simulink model "MPCwithStage"  (R2019b)
settings: Solver=ode8  StartTime=0.0  StopTime=5  RelTol=1e-3
settings Model: Creator=cwh  LastModifiedBy=cwh

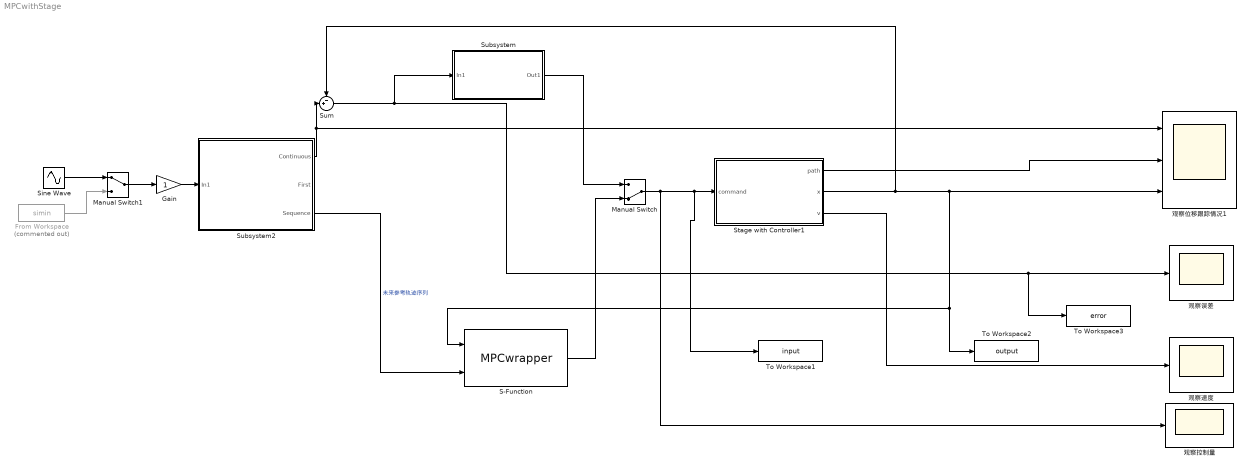
== system MPCwithStage ==
  From Workspace : FromWorkspace  Commented=on  VariableName=simin
  Gain : Gain
  Manual Switch : ManualSwitch  CurrentSetting=0
  Manual Switch1 : ManualSwitch
  S-Function : S-Function  FunctionName=MPCwrapper  Parameters=ts0,p0,m0,wy0,wu0,pn0,mn0,A0,B0,C0  SFunctionDeploymentMode=off  EnableBusSupport=off  mask{ts0=1/300, p0=15, m0=2, wy0=1, wu0=2, pn0=0.01, mn0=1e-7, A0=[1.00001139444525 0.000608242190743377;-0.00132825987534539 0.740443856051726], B0=[0.00434874017606072;-35.613687675832], C0=[-6.04865289015463 -0.00170156787433402]}
      mask Display:
      | fprintf('MyMPCinC++');
      | port_label('input', 1, 'mo')
      | port_label('input', 2, 'ref')
      | port_label('output', 1, 'mv')
  Sine Wave : Sin  Amplitude=0.001  Frequency=2*3.1415926*2  SampleTime=0
  Stage with Controller1 : Subsystem  mask{tc=1/300, ts=5e-5, vm=0.5, am=3}
      mask prompts: tc "Command period"; ts "Servoing period"; vm "vmax"; am "amax"
  Subsystem : Subsystem  mask{kp=2, ki=0, kd=0.01}
      mask Display:
      | fprintf('PID Controller');
      | port_label('input', 1, 'error')
      | port_label('output', 1, 'out')
  Subsystem2 : Subsystem  mask{tc=1/300, p=15}
      mask prompts: tc "Control period"; p "Preview Length"
  Sum : Sum  Inputs=-+|
  To Workspace1 : ToWorkspace  VariableName=input  SampleTime=1/300
      settings: Save2DSignal=2-D array (concatenate along first dimension)
  To Workspace2 : ToWorkspace  VariableName=output  SampleTime=1/300
      settings: Save2DSignal=2-D array (concatenate along first dimension)
  To Workspace3 : ToWorkspace  VariableName=error  SampleTime=1/300
      settings: Save2DSignal=2-D array (concatenate along first dimension)
  观察位移跟踪情况1 : Scope  NumInputPorts=3
  观察控制量 : Scope
  观察误差 : Scope
  观察速度 : Scope
  wires:
  S-Function/1 -> Manual Switch/2
  From Workspace/1 -> Manual Switch1/2
  Gain/1 -> Subsystem2/1(In1)
  Manual Switch1/1 -> Gain/1
  Sine Wave/1 -> Manual Switch1/1
  Subsystem2/3(Sequence) -> S-Function/2  "未来参考轨迹序列"
  Manual Switch/1 -> Stage with Controller1/1(command), To Workspace1/1, 观察控制量/1
  Stage with Controller1/2(x) -> Sum/1, S-Function/1, To Workspace2/1, 观察位移跟踪情况1/3
  Sum/1 -> To Workspace3/1, 观察误差/1, Subsystem/1(In1)
  Stage with Controller1/1(path) -> 观察位移跟踪情况1/2
  Subsystem/1(Out1) -> Manual Switch/1
  Stage with Controller1/3(v) -> 观察速度/1
  Subsystem2/1(Continuous) -> 观察位移跟踪情况1/1, Sum/2

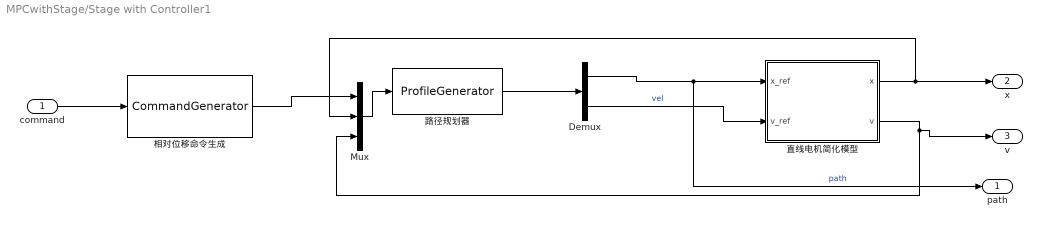
== system MPCwithStage/Stage with Controller1 ==
  command : Inport
  Demux : Demux  Outputs=2
  Mux : Mux  Inputs=3
  直线电机简化模型 : Subsystem  mask{ts=ts, L=1.94e-3, R=2.46, Ki=4.6, Kf=0, Kbemf=2.81, M=1, Kpx=15, Kix=0.001, Kdx=0.02, Kpv=0.05, Kiv=0.5, Kdv=0, Kpi=5, Kii=0.0015, Kdi=0}
      mask prompts: ts "Servoing period"; L "Coil inductance"; R "Coil resistance"; Ki "Force coefficient"; Kf "Friction coefficient"; Kbemf "Back EMF Coefficient"; M "Moving mass"; Kpx "Kp in position loop"; Kix "Ki in position loop"; Kdx "Kd in position loop"; Kpv "Kp in velocity loop"; Kiv "Ki in velocity lpop"; Kdv "Kd in velocity loop"; Kpi "Kp in current loop"; Kii "Ki in current loop"; Kdi "Kd in current loop"
  相对位移命令生成 : S-Function  FunctionName=CommandGenerator  Parameters=ts0,cp0  SFunctionDeploymentMode=off  EnableBusSupport=off  mask{ts0=ts, cp0=tc}
      mask prompts: ts0 "Serving period"; cp0 "Command period"
  路径规划器 : S-Function  FunctionName=ProfileGenerator  Parameters=ts0,vmax0,amax0  SFunctionDeploymentMode=off  EnableBusSupport=off  mask{ts0=ts, vmax0=vm, amax0=am}
      mask prompts: ts0 "Servoing period"; vmax0 "Max velocity"; amax0 "Max acceleration"
  path : Outport
  x : Outport  Port=2
  v : Outport  Port=3
  wires:
  Demux/2 -> 直线电机简化模型/2(v_ref)  "vel"
  Demux/1 -> path/1, 直线电机简化模型/1(x_ref)  "path"
  直线电机简化模型/1(x) -> x/1, Mux/2
  command/1 -> 相对位移命令生成/1
  Mux/1 -> 路径规划器/1
  路径规划器/1 -> Demux/1
  相对位移命令生成/1 -> Mux/1
  直线电机简化模型/2(v) -> v/1, Mux/3

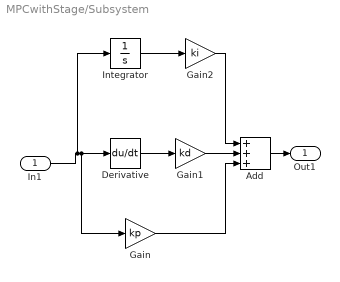
== system MPCwithStage/Subsystem ==
  In1 : Inport
  Add : Sum  Inputs=+++
  Derivative : Derivative
  Gain : Gain  Gain=kp
  Gain1 : Gain  Gain=kd
  Gain2 : Gain  Gain=ki
  Integrator : Integrator
  Out1 : Outport
  wires:
  In1/1 -> Integrator/1, Gain/1, Derivative/1
  Integrator/1 -> Gain2/1
  Derivative/1 -> Gain1/1
  Gain2/1 -> Add/1
  Gain1/1 -> Add/2
  Gain/1 -> Add/3
  Add/1 -> Out1/1

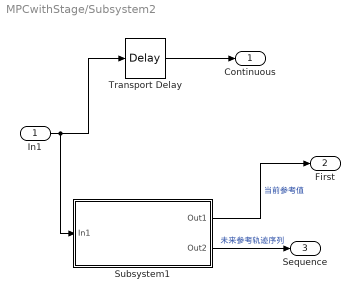
== system MPCwithStage/Subsystem2 ==
  In1 : Inport
  Subsystem1 : Subsystem  mask{ts0=tc, length0=p}
      mask prompts: ts0 "Sample time"; length0 "Preview length"
      mask Display:
      | fprintf('Reference\nPreviewer');
      | port_label('input', 1, 'input')
      | port_label('output', 1, 'first')
      | port_label('output', 2, 'seq')
  Transport Delay : TransportDelay  DelayTime=tc*p
  Continuous : Outport
  First : Outport  Port=2
  Sequence : Outport  Port=3
  wires:
  In1/1 -> Subsystem1/1(In1), Transport Delay/1
  Transport Delay/1 -> Continuous/1
  Subsystem1/1(Out1) -> First/1  "当前参考值"
  Subsystem1/2(Out2) -> Sequence/1  "未来参考轨迹序列"

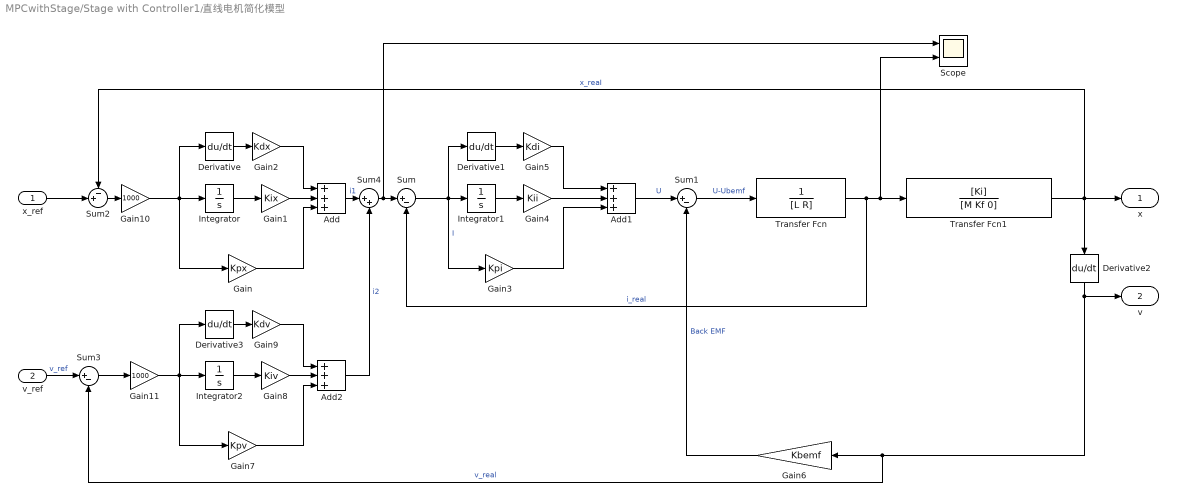
== system MPCwithStage/Stage with Controller1/直线电机简化模型 ==
  x_ref : Inport
  v_ref : Inport  Port=2
  Add : Sum  Inputs=+++
  Add1 : Sum  Inputs=+++
  Add2 : Sum  Inputs=+++
  Derivative{,1..3} (4 alike) : Derivative
  Gain : Gain  Gain=Kpx
  Gain1 : Gain  Gain=Kix
  Gain10 : Gain  Gain=1000
  Gain11 : Gain  Gain=1000
  Gain2 : Gain  Gain=Kdx
  Gain3 : Gain  Gain=Kpi
  Gain4 : Gain  Gain=Kii
  Gain5 : Gain  Gain=Kdi
  Gain6 : Gain  Gain=Kbemf
  Gain7 : Gain  Gain=Kpv
  Gain8 : Gain  Gain=Kiv
  Gain9 : Gain  Gain=Kdv
  Integrator : Integrator
  Integrator1 : Integrator
  Integrator2 : Integrator
  Scope : Scope  NumInputPorts=2
  Sum : Sum  Inputs=|+-
  Sum1 : Sum  Inputs=|+-
  Sum2 : Sum  Inputs=-+|
  Sum3 : Sum  Inputs=|+-
  Sum4 : Sum  Inputs=|++
  Transfer Fcn : TransferFcn  Denominator=[L R]
  Transfer Fcn1 : TransferFcn  Numerator=[Ki]  Denominator=[M Kf 0]
  x : Outport
  v : Outport  Port=2
  wires:
  Gain10/1 -> Derivative/1, Gain/1, Integrator/1
  Derivative/1 -> Gain2/1
  Integrator/1 -> Gain1/1
  Gain2/1 -> Add/1
  Gain1/1 -> Add/2
  Gain/1 -> Add/3
  Sum/1 -> Derivative1/1, Gain3/1, Integrator1/1  "I"
  Gain3/1 -> Add1/3
  Gain4/1 -> Add1/2
  Integrator1/1 -> Gain4/1
  Gain5/1 -> Add1/1
  Derivative1/1 -> Gain5/1
  Add1/1 -> Sum1/1  "U"
  Transfer Fcn/1 -> Scope/2, Transfer Fcn1/1, Sum/2  "i_real"
  Sum1/1 -> Transfer Fcn/1  "U-Ubemf"
  Transfer Fcn1/1 -> x/1, Sum2/1, Derivative2/1  "x_reaI"
  Derivative2/1 -> v/1, Sum3/2, Gain6/1  "v_real"
  Gain6/1 -> Sum1/2  "Back EMF"
  Gain7/1 -> Add2/3
  Gain11/1 -> Derivative3/1, Gain7/1, Integrator2/1
  Gain8/1 -> Add2/2
  Integrator2/1 -> Gain8/1
  Add2/1 -> Sum4/2  "i2"
  Gain9/1 -> Add2/1
  Derivative3/1 -> Gain9/1
  v_ref/1 -> Sum3/1  "v_ref"
  Add/1 -> Sum4/1  "i1"
  Sum4/1 -> Scope/1, Sum/1
  x_ref/1 -> Sum2/2
  Sum3/1 -> Gain11/1
  Sum2/1 -> Gain10/1

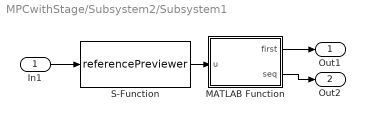
== system MPCwithStage/Subsystem2/Subsystem1 ==
  In1 : Inport
  MATLAB Function : MATLAB Function  TreatAsAtomicUnit=on
  S-Function : S-Function  FunctionName=referencePreviewer  Parameters=ts0,length0  SFunctionDeploymentMode=off  EnableBusSupport=off
  Out1 : Outport  VectorParamsAs1DForOutWhenUnconnected=off
  Out2 : Outport  Port=2  VectorParamsAs1DForOutWhenUnconnected=off
  wires:
  MATLAB Function/1(first) -> Out1/1
  MATLAB Function/2(seq) -> Out2/1
  S-Function/1 -> MATLAB Function/1(u)
  In1/1 -> S-Function/1

== matlab function MPCwithStage/Subsystem2/Subsystem1/MATLAB Function ==
  data: u input; first output; seq output
function [first,seq]= fcn(u)
seq=u(2:max(size(u)));
first=u(1);
